simulink model "discretka"  (R2021b)
settings: Solver=VariableStepAuto  StartTime=0.0  StopTime=0.3  RelTol=1e-3
settings Model: Creator=snipe  LastModifiedBy=snipe

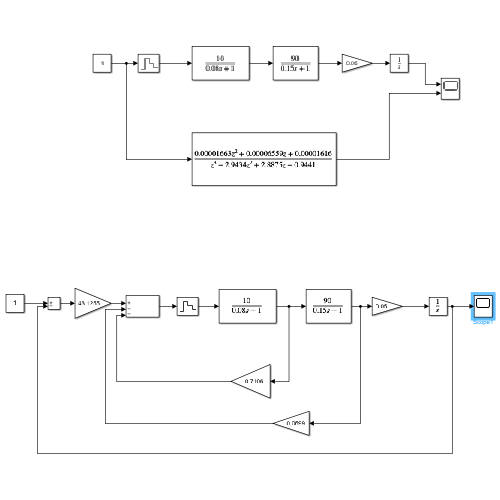
[thumbnail: Simulink's stored preview of the top-level diagram]
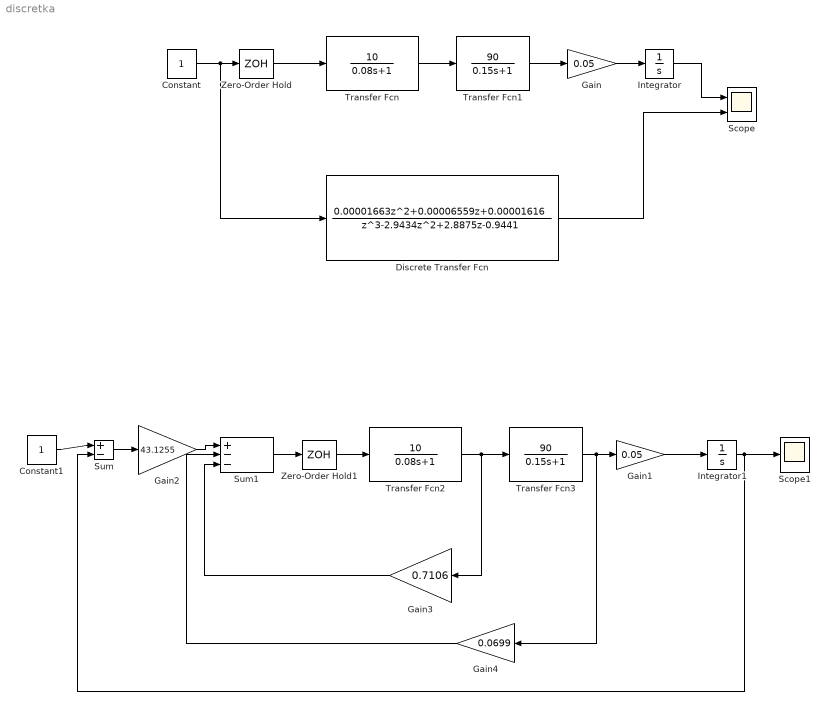
== system discretka ==
  Constant : Constant
  Constant1 : Constant
  Discrete Transfer Fcn : DiscreteTransferFcn  Numerator=[0 0.00001663 0.00006559 0.00001616]  Denominator=[1 -2.9434 2.8875 -0.9441]
  Gain : Gain  Gain=0.05
  Gain1 : Gain  Gain=0.05
  Gain2 : Gain  Gain=43.1255
  Gain3 : Gain  Gain=0.7106
  Gain4 : Gain  Gain=0.0699
  Integrator : Integrator
  Integrator1 : Integrator
  Scope : Scope  NumInputPorts=2
  Scope1 : Scope
  Sum : Sum  Inputs=|+-
  Sum1 : Sum  Inputs=|+--
  Transfer Fcn : TransferFcn  Numerator=[0 10]  Denominator=[0.08 1]
  Transfer Fcn1 : TransferFcn  Numerator=[90]  Denominator=[0.15 1]
  Transfer Fcn2 : TransferFcn  Numerator=[0 10]  Denominator=[0.08 1]
  Transfer Fcn3 : TransferFcn  Numerator=[90]  Denominator=[0.15 1]
  Zero-Order Hold : ZeroOrderHold  SampleTime=-1
  Zero-Order Hold1 : ZeroOrderHold  SampleTime=-1
  wires:
  Constant/1 -> Discrete Transfer Fcn/1, Zero-Order Hold/1
  Zero-Order Hold/1 -> Transfer Fcn/1
  Transfer Fcn/1 -> Transfer Fcn1/1
  Transfer Fcn1/1 -> Gain/1
  Gain/1 -> Integrator/1
  Integrator/1 -> Scope/1
  Discrete Transfer Fcn/1 -> Scope/2
  Transfer Fcn3/1 -> Gain4/1, Gain1/1
  Transfer Fcn2/1 -> Gain3/1, Transfer Fcn3/1
  Gain1/1 -> Integrator1/1
  Zero-Order Hold1/1 -> Transfer Fcn2/1
  Constant1/1 -> Sum/1
  Sum1/1 -> Zero-Order Hold1/1
  Integrator1/1 -> Scope1/1, Sum/2
  Sum/1 -> Gain2/1
  Gain2/1 -> Sum1/1
  Gain4/1 -> Sum1/2
  Gain3/1 -> Sum1/3
